simulink model "ADU_Integration_Y2016_simulation"  (R2016b)
settings: Solver=FixedStepDiscrete  StartTime=240  StopTime=300  FixedStep=0.01  RelTol=1e-3  EnableMultiTasking=on
PostLoadFcn:
  | , if any(exist('dsrtsu_mdlpostloadfcn', 'file') == [2, 3, 6]), try dsrtsu_mdlpostloadfcn('Execute', bdroot); catch fprintf('Error in PostLoadFcn (dsrtsu_mdlpostloadfcn) for model "%s":\n %s\n', bdroot, lasterr); end, end,
InitFcn:
  | load 'data/chi2_dat';
  | load 'data/innerLine_struct';
  | load 'data/middleLine_struct';
  | load 'data/outerLine_struct';
  | load 'data/innerLine';
  | load 'data/middleLine';
  | load 'data/outerLine';
  | load 'data/landmarks_patac_schimmel_ccw';
  | load 'data/patac_navi_array';
  | load 'data/sensor';
  | load 'data/map_struct';
  | addpath map_src
  | Integration_Parameter;
  | load 'TestData_001';
values from neighbouring files (symbols this model uses):
  TestData_001 =     [TestData_001.mat]
undefined symbols (not defined in the file or in its folder): a, chi2_dat, innerLine, landmarks_patac_schimmel_ccw, middleLine, outerLine, patac_navi_array, StartNum
libraries: simulink x36, rtican x1
(part 19 of 20)

== matlab function ADU_Integration_Y2016_simulation/Path_Plan1/LaneChangePathPlanningModule1/PathCreator/PathCreator ==
  data: xoptres output; Info_FdIn input; Info_FoIn input; Info_LdIn input; Info_LoIn input; Info_MeIn input; PlanRes output; Tc data_store_memory; V_me data_store_memory; V data_store_memory; L_veh data_store_memory; X_me data_store_memory; X data_store_memory; L_me data_store_memory; T_adj data_store_memory; H data_store_memory; AngleTC data_store_memory; Y data_store_memory; W_veh data_store_memory; Y_me data_store_memory; W_me data_store_memory; Aylimit data_store_memory; Axlimit data_store_memory; X_melimit data_store_memory; k_maxlimit data_store_memory; MSS data_store_memory; DeltaTemp data_store_memory; ArclengthTol data_store_memory; x_qitemp data_store_memory; y_qitemp data_store_memory; theta_qitemp data_store_memory; k_localmaxTemp data_store_memory; ploten data_store_memory; ratio data_store_memory; N_Sample data_store_memory; quadcosu2tbl data_store_memory; quadsinu2tbl data_store_memory; x_inIn input; y_inIn input; angle_inIn input; y_outIn input; angle_outIn input; T_lat data_store_memory; x_in data_store_memory; y_in data_store_memory; angle_in data_store_memory; angle_out data_store_memory; y_out data_store_memory; KurMax output; TrigFlg input; X_melimit_In input; N input; Nlimit data_store_memory; RunCnt data_store_memory; N2 input; Nlimit2 data_store_memory
function [xoptres,PlanRes,KurMax] = PathCreatorFcn(Info_FdIn,Info_FoIn,Info_LdIn,Info_LoIn,Info_MeIn,x_inIn,y_inIn,angle_inIn,y_outIn,angle_outIn,TrigFlg,X_melimit_In,N,N2)
%     global Aylimit Axlimit X_melimit k_maxlimit Tc V L_veh  X L_me T_adj H AngleTC  Y W_veh  W_me X_me MSS x_qitemp y_qitemp theta_qitemp;
    global T_lat V_me DeltaTemp ArclengthTol k_localmaxTemp Nlimit Nlimit2 
    persistent TrigCnt FinishFlg
    if isempty(TrigCnt)
        TrigCnt = 0;
    end
    if isempty(FinishFlg)
        FinishFlg = 1;
    end    
    Nlimit = N;
    Nlimit2 = N2;

    xoptres = [0 0 0]';PlanRes = 0; KurMax = 0;T_long = 4; 
    PreGlbVal(x_inIn,y_inIn,angle_inIn,y_outIn,angle_outIn,Info_FdIn,Info_FoIn,Info_LdIn,Info_LoIn,Info_MeIn,X_melimit_In);
    %Edge Trigger
    if (TrigFlg > 1e-1)
        FinishFlg = 0;
    end
    if FinishFlg == 0
        LB = [10,0.1,5];UB = [40,0.5,20];x0 = [20,0.4,10];
        TrigCnt = 1;
        [xoptres,Res,Sts] = SQPCal(x0',LB',UB',TrigCnt);
        if Sts == 1
            FinishFlg = 1;
            if Res == 1
                PlanRes = 1;  TrigCnt = 0;
%                 x_out=xoptres(1);
%                 V_tar=xoptres(3);
%                 S_arc = ArclengthTol(1) + ArclengthTol(2);    
%                 T_long=xoptres(2)*2*S_arc/(V_tar + V_me);
%                 S_acc = (V_tar + V_me)/2 * T_long;
%                 S_arc = ArclengthTol(1) + ArclengthTol(2);
%                 if S_acc < S_arc
%                     T_lat = T_long + (S_arc - S_acc) / V_tar;
%                 else
%                     a = (V_tar - V_me)/T_long;
%                     V_end = sqrt(V_me^2 + 2*a*S_arc);
%                     if a == 0
%                         T_lat = S_arc / V_me;
%                     else        
%                         T_lat = (V_end - V_me)/a;
%                     end
%                 end 
%                 [ x_qi,y_qi,theta_qi ] = qiConfigCal( x_inIn,y_inIn,angle_inIn,x_out,y_outIn,angle_outIn );
%                 [DeltaTemp(1),k_localmaxTemp(1),ArclengthTol(1)] = ElementaryPathPlot( x_inIn,y_inIn,angle_inIn,x_qi,y_qi,theta_qi );
%                 [DeltaTemp(2),k_localmaxTemp(2),ArclengthTol(2)] = ElementaryPathPlot( x_qi,y_qi,theta_qi,x_out,y_outIn,angle_outIn );
                KurMax = max(k_localmaxTemp);
            end
        else
            TrigCnt = TrigCnt + 1;
        end
    end  
end

function [xoptim,Res,Sts] = SQPCal(x0,LB,UB,Trig)

    global ratio
    global Nlimit Nlimit2
    persistent FinishFlg Pdk PLamda Px1 PCostGTemp PConGTemp StepTrigFlg RunCnt PHk PBk PCurStep PCostG PConG PHx 
    if isempty(RunCnt)
        RunCnt = 0;
    end
    if isempty(PHk)   
        PHk = eye(3);
    end
    if isempty(PBk)   
        PBk = eye(3);
    end    
    if isempty(FinishFlg)
        FinishFlg = 0;
    end
    if isempty(Pdk)
        Pdk = [1 1 1]';
    end
    if isempty(PLamda)
        PLamda = ones(14,1);
    end
    if isempty(Px1)
        Px1 = x0;
    end
    if isempty(PCostGTemp)
        PCostGTemp = zeros(3,1);
    end
    if isempty(PConGTemp)
        PConGTemp = zeros(3,14);
    end
    if isempty(StepTrigFlg)
        StepTrigFlg = 0;
    end
    if isempty(PCurStep)
        % 1 golden 2 qpsub
        PCurStep = 1;
    end
    if isempty(PCostG)
        PCostG = zeros(3,1);
    end
    if isempty(PConG)
        PConG = zeros(3,14);
    end
    if isempty(PHx)
        PHx = zeros(1,14);
    end
    ratio = 1e3;
    limit1 = [0 0 0];limit2 = [0 0 0];lolimit = [0 0 0];hilimit = [0 0 0]; Alpha = 1;
    dk = [1 1 1]'; Lamda = ones(14,1);  x1 = x0;Bk=eye(3);Hk=eye(3);xoptim = x0;; CostGTemp = zeros(3,1);ConGTemp = zeros(3,14);Sts = 0;Res = 0;CostG = zeros(3,1);ConG = zeros(3,14);Hx = zeros(1,14);
%     while (1)
    if PCurStep == 1
        if (RunCnt == 0)
            if Trig == 1
                %First Trig 
                RunCnt = RunCnt + 1;
                FinishFlg = 0;
                [CostG,ConG,Costx,Hx]=GradientCal(x0,LB,UB);
                CostGTemp = CostG;
                ConGTemp = ConG;
            end
        else
            %LoadFrom Previous Step
            dk = Pdk;Lamda = PLamda;x1 = Px1;CostGTemp = PCostGTemp;ConGTemp = PConGTemp;Hk = PHk;Bk = PBk;
            for i = 1:3
                if abs(dk(i)) < 1e-4
                    limit1(i) = 0;
                    limit2(i) = 1e4;                
                else
                    limit1(i) = ((LB(i) - x1(i))./dk(i));
                    limit2(i) = ((UB(i) - x1(i))./dk(i));
                end
                lolimit(i) = min([limit1(i),limit2(i)]);
                hilimit(i) = max([limit1(i),limit2(i)]);
            end
            Lo = max([lolimit,0]);
            Hi = min(hilimit);
            if (Hi <0)||(Hi < Lo)
                FinishFlg = 1;
            end
            Accurcy = min(abs([1e-2/dk(1),1e-3/dk(2),1e-2/dk(3)]));
            Alpha=goldenSearch(x1,dk,Lo,Hi,LB,UB,Accurcy);
            if max(abs(Alpha * dk)) < 1e-3
                FinishFlg = 1;
            end
            BestStep = Alpha * dk;
            if (BestStep(1) < 1e-2)&& (BestStep(3) < 1e-2) && (BestStep(2) < 1e-3)                          
            end
            x1temp = x1;
            x1 = x1 + Alpha * dk;
            sk=x1-x1temp; 
            [CostG,ConG,Costx,Hx] = GradientCal(x1,LB,UB);
            initial_CostGLx = LxGradientCal(CostGTemp,ConGTemp,Lamda);
            CostGLx = LxGradientCal(CostG,ConG,Lamda);
            CostGTemp = CostG;
            ConGTemp = ConG;
            yk = CostGLx-initial_CostGLx; 
            if  yk'*sk>0
                Bk=Bk+(sk*sk')/(yk'*sk)-(Bk*yk*yk'*Bk)/(yk'*Bk*yk);  
            else 
            end
            if yk'* sk > 0 
                Hk = Hk + ((sk - Hk*yk)*sk' + sk*(sk-Hk*yk)')/(yk'*sk)-(sk-Hk*yk)'*yk*sk*sk'/(yk'*sk)^2;
            end
        end
        PHk = Hk;PCostG = CostG;PConG = ConG;PHx = Hx;Px1 = x1;PConGTemp = ConGTemp;PBk = Bk;PCostGTemp = CostGTemp; 
        PCurStep = 2;
    else          
        if (FinishFlg == 0)&&(PCurStep == 2)
            Hk = PHk;CostG = PCostG;ConG = PConG;Hx = PHx;PCurStep = 1;
            y1 = ones(14,1);w1 = ones(14,1);dx1 = ones(3,1);
            [dk,Lamda] = qpfunc( Hk,CostG,ConG',-Hx,dx1,y1,w1 );  
            if (norm(dk,2)<1e-3)||(Alpha < 1e-4)
                FinishFlg = 1;
            else
                Pdk = dk; PLamda = Lamda; 
            end
        end
        PCurStep = 1; 
    end
    RunCnt = RunCnt + 1;
    if RunCnt > Nlimit
        FinishFlg = 1;
    end
    if FinishFlg == 1;        
        Sts = 1;
        if RunCnt > Nlimit
            % 0 Failure 1 Success
           Res = 0;
        else
           Res = 1;
           xoptim = Px1; 
        end
        RunCnt = 0;PCurStep = 1;
    end
end

function [CostG,ConG,Costx,Hx]= GradientCal(Xin,LB,UB)

value1Cost=ones(3,1);
value2Cost=ones(3,1);
value1Con=ones(3,14);
value2Con=ones(3,14);

dx=1e-1;
dy=1e-1;
dz=1e-1;
Xin_x=Xin+ [dx;0;0];
Xin_y=Xin+ [0;dy;0];
Xin_z=Xin+ [0;0;dz];
value1Cost(1) = (  CostFun(Xin_x) - CostFun(Xin) ) / dx;    %x
value1Cost(2) = (  CostFun(Xin_y) - CostFun(Xin) ) / dy ;   %y
value1Cost(3) = (  CostFun(Xin_z) - CostFun(Xin) ) / dz ;   %z
ConFuncXinVal = ConFunc(Xin,LB,UB);
value1Con(1,:) = (  ConFunc(Xin_x,LB,UB) - ConFuncXinVal ) / dx;    %x
value1Con(2,:) = (  ConFunc(Xin_y,LB,UB) - ConFuncXinVal ) / dy ;   %y
value1Con(3,:) = (  ConFunc(Xin_z,LB,UB) - ConFuncXinVal ) / dz ;   %z
CostG = value1Cost;
ConG = value1Con;
Costx = CostFun(Xin);
Hx = ConFuncXinVal;

end

function bestStep=goldenSearch(x0,direction,lo,hi,LB,UB,Accurcy)
    global Nlimit 
    a=lo;
    b=hi;
    % TBD Change 2
    error=1e-2;
    error = Accurcy;
    golden=0.61803398;
    goldenn = 0;
    alpha=a + (1-golden) * (b-a);
    beta=a + golden * (b-a);
    f_alpha=Pfunc( x0 + alpha * direction,LB,UB);
    f_beta=Pfunc( x0 + beta * direction,LB,UB);

    while(abs(b-a)>error)

    %     a1=a;  b1=b;
        goldenn = goldenn + 1;
        b - a;
        f_beta - f_alpha;
        if alpha>beta
    %         a=a1;b=b1;
            alpha=a + (1-golden) * (b-a);
            beta=a + golden * (b-a);
            f_alpha=Pfunc( x0 + alpha * direction,LB,UB);
            f_beta=Pfunc( x0 + beta * direction,LB,UB);       
        end  
        if f_alpha<=f_beta
            b=beta;
            beta=alpha;
            f_beta=f_alpha;
            alpha=a + (b-beta);
            f_alpha=Pfunc( x0 + alpha*direction,LB,UB);
    %         a1=a;  b1=b;
        else
            a = alpha;
            alpha = beta;
            f_alpha = f_beta;
            beta = b - (alpha-a);
            f_beta = Pfunc( x0 + beta * direction,LB,UB);
    %         a1=a;  b1=b;
        end
        if goldenn > Nlimit
            break;
        end

    end

    if Pfunc(x0 + a * direction,LB,UB)<Pfunc(x0 + b * direction,LB,UB)
        bestStep=a;
    else
        bestStep=b;
    end
    n = 0;
    goldenn
end

function [dk,dkLamda] = qpfunc( H,c,A,b,x1,y1,w1 )
%UNTITLED2 Summary of this function goes here
%   Detailed explanation goes here
    global Nlimit 
Delta = 0.1;
P = 0.9;
E = ones(length(y1),1);
m = length(b);
qpfunck = 0;

    while(1)

        qpfunck = qpfunck+1;
        if qpfunck > Nlimit
            dk = x1;
            dkLamda = y1;
            break;
        end
        Y = diag(y1);
        W = diag(w1);
        Rho = b - A*x1 + w1;
        Sigma = c + H*x1 -A'*y1;
        Gamma = y1'*w1;
        Mu = Delta * Gamma / m;
        newMatricL = [-H A';A inv(Y)*W];
        newMatricR = [c + H*x1 - A'*y1;b-A*x1 + Mu*inv(Y)*E];
        dxy = inv(newMatricL)*newMatricR;
        dx = dxy(1:length(x1));
        dy = dxy((length(x1)+1):(length(dxy)));
        dw = inv(Y)*(Mu*E - Y*W*E - W*dy);
        LamdaTemp1 = [-dy./y1,-dw./w1];
        Lamda = min([1, P*pinv(max([-dy./y1;-dw./w1]))]);
        if (norm(Gamma,1)<1e-3)&(norm(Rho,1)<1e-3)&(norm(Sigma,1)<1e-3)
            dk = x1;
            dkLamda = y1;
            break;
        else
            x1 = x1 + Lamda*dx;
            y1 = y1 + Lamda*dy;
            w1 = w1 + Lamda*dw;
        end
    end
    qpfunck;
end

function dLxVal= LxGradientCal2(Xin,Lamda,LB,UB,CostGTemp,ConGTemp)

    value1=ones(3,1);
    value2=ones(3,1);
    value1LxVal = [0 0 0];
    value2LxVal = [0 0 0];
    dx=1e-1;
    dy=1e-1;
    dz=1e-1;
    Xin_x=Xin+ [dx;0;0];
    Xin_y=Xin+ [0;dy;0];
    Xin_z=Xin+ [0;0;dz];

    ConFuncValue = ConFunc(Xin,LB,UB);

    value1LxVal(1) = (CostFun(Xin_x) - CostFun(Xin)- Lamda' *  ConFunc(Xin_x,LB,UB) + Lamda' *  ConFuncValue)/dx;
    value1LxVal(2) = (CostFun(Xin_y) - CostFun(Xin)- Lamda' *  ConFunc(Xin_y,LB,UB) + Lamda' *  ConFuncValue)/dy;
    value1LxVal(3) = (CostFun(Xin_z) - CostFun(Xin)- Lamda' *  ConFunc(Xin_z,LB,UB) + Lamda' *  ConFuncValue)/dz;

    dLxVal = value1LxVal;
    dLxVal = dLxVal';
    
end
% TBD change 5

function dLxVal= LxGradientCal(CostG,ConG,Lamda)

    dLxVal = CostG -  ConG* Lamda;
    
end

function Pval= Pfunc(Xin,LB,UB)
    global ratio   
    [C,Ceq] = LaneChgNonLinearCon( Xin);
    LengthC = 8;
    LengthLB = length(LB);
    C((LengthC+1):(LengthC+LengthLB))= Xin - UB;
    C((LengthC+LengthLB+1):(LengthC+LengthLB+LengthLB))= LB - Xin;

    hminx= min([0,min(-C)]);
    Pval = - Xin(3) + ratio* norm(hminx,1);
end

function Fcost= CostFun(Xin)

    Fcost = LaneChgCostFunc(Xin);

end

function ConVal= ConFunc(Xin,LB,UB)
    [C,Ceq] = LaneChgNonLinearCon( Xin);

    LengthC = 8;
    LengthLB = length(LB);
    C((LengthC+1):(LengthC+LengthLB))= Xin - UB;
    C((LengthC+LengthLB+1):(LengthC+LengthLB+LengthLB))= LB - Xin;
    C=-C;
    ConVal = C;

end
function CosFunValue = LaneChgCostFunc(Xin)
    CosFunValue = -Xin(3);
end
function [ C,Ceq ] = LaneChgNonLinearCon( Xin )
global V_me V L_veh X_me X L_me T_adj ;
global Aylimit  X_melimit k_maxlimit;
% global T_lat Axlimit 
global DeltaTemp k_localmaxTemp ArclengthTol
global x_qitemp y_qitemp theta_qitemp
global x_in y_in angle_in y_out angle_out 
C = zeros(14,1);
Tc = [0 0 0 0]';
MSS = [0 0 0 0]';
%T_long=Xin(2);
V_tar=Xin(3);

T_lat = 5;
% x_in = 0;y_in = 0;angle_in = 0;y_out = 3;angle_out = 0;
x_out = Xin(1);
[ x_qi,y_qi,theta_qi ] = qiConfigCal( x_in,y_in,angle_in,x_out,y_out,angle_out );
 x_qitemp = x_qi;y_qitemp=y_qi;theta_qitemp=theta_qi;
%[ x_qitemp,y_qitemp,theta_qitemp ] = qiConfigCal( x_in,y_in,angle_in,x_out,y_out,angle_out );
[DeltaTemp(1),k_localmaxTemp(1),ArclengthTol(1)] = ElementaryPathPlot( x_in,y_in,angle_in,x_qi,y_qi,theta_qi );
[DeltaTemp(2),k_localmaxTemp(2),ArclengthTol(2)] = ElementaryPathPlot( x_qi,y_qi,theta_qi,x_out,y_out,angle_out );
Ycal = [1.5,1.5];
% 1 Fl 2 Rr
[xposition,yposition,Theta,ArcPos] = ArcPosCal( angle_out,angle_in,x_in,y_in,x_out,y_out,Ycal );
%Fd
Tc(1) = (xposition(1) - X(1))/(V(1)+1e-6);
Tc(2) = (xposition(2) - X(2))/(V(2)+1e-6);
Tc(3) = (xposition(1) - X(3))/(V(3)+1e-6);
Tc(4) = (xposition(2) - X(4))/(V(4)+1e-6);
for i = 1:4
    if Tc(i) < 0
        Tc(i) = 0;
    else
    end
end
        
delta_limit = 0.5;
DeltalimitC = max(abs(DeltaTemp)) - delta_limit;
AylimitC = max(abs(k_localmaxTemp)) * V_tar^2 - Aylimit;
KmlimitC = max(abs(k_localmaxTemp)) - k_maxlimit;

S_arc = ArclengthTol(1) + ArclengthTol(2);
if V_tar == V_me
    T_lat = S_arc / V_me;
    T_long = 0;
else
    Tuplimit = 2 * S_arc / (V_tar + V_me);
    T_long = Tuplimit * Xin(2);
    S_acc = (V_tar + V_me)/2 * T_long;
    if S_acc < S_arc
        T_lat = T_long + (S_arc - S_acc) / V_tar;
    else
        a = (V_tar - V_me)/T_long;
        V_end = sqrt(V_me^2 + 2*a*S_arc);
        if a == 0
            T_lat = S_arc / V_me;
        else        
            T_lat = (V_end - V_me)/a;
        end
    end
end
%MSSFdlimitC < 0 which means safemargin >0
MSS(1) = MSSFdJudgment( V_tar,V_me,V(1),T_lat,Tc(1),T_lat,T_adj );
MSS(2) = MSSFoJudgment( V_tar,V_me,V(2),T_lat,Tc(2),T_lat,T_adj );
MSS(3) = MSSLdJudgment( V_tar,V_me,V(3),T_lat,Tc(3),T_lat,T_adj );
MSS(4) = MSSLoJudgment( V_tar,V_me,V(4),T_lat,Tc(4),T_lat,T_adj );
X_meTemp = X_me - 2 * (ArcPos(1)+ArcPos(2) - xposition(1) - xposition(2));
MSSFdlimitC = X(1) - X_meTemp + L_me + MSS(1);
MSSFolimitC = X(2) - X_meTemp + L_me + MSS(2);
MSSLdlimitC = MSS(3) + X_meTemp + L_veh(3) - X(3);
MSSLolimitC = MSS(4) + X_meTemp + L_veh(4) - X(4);
X_melimitC =  2 * x_out - X_melimit;

C(1)=DeltalimitC;
C(2)=KmlimitC;
C(3)=MSSFdlimitC;
C(4)=MSSFolimitC;
C(5)=MSSLdlimitC;
C(6)=MSSLolimitC;
C(7)=X_melimitC;
C(8)=AylimitC; 

Ceq = [];

end

function [xposition,yposition,Theta,ArcPos] = ArcPosCal( angle_out,angle_in,x_in,y_in,x_out,y_out,Ycal )
%UNTITLED2 Summary of this function goes here
%   Detailed explanation goes here
    global  ArclengthTol
%     global x_qitemp y_qitemp theta_qitemp k_localmaxTemp DeltaTemp
    xposition = [0 0];
    yposition = [1.5 1.5];
    Theta = [0 0 ];
    ArcPos = [0 0];
    [ArcPos,xposition,Theta] = SecantMethod2( angle_out,angle_in,x_in,y_in,x_out,y_out,0.8*ArclengthTol(1),1.1*ArclengthTol(1) ); 
end
 
% end
function [xres,xposition,theta] = SecantMethod2( angle_out,angle_in,x_in,y_in,x_out,y_out,x0,x1 )
    xres = [0 0 ];
    temp1 = x0;
    temp2 = x1;
    xposition = [0 0];
    theta = [0 0]; 
    [xpositionFl1,ypositionFl1,ThetaFl1] = LaneChgFlPosCal2( x1,angle_out,angle_in,x_in,y_in,x_out,y_out );
    funx1 = ypositionFl1 - 1.5;
    [xpositionFl0,ypositionFl0,ThetaFl0] = LaneChgFlPosCal2( x0,angle_out,angle_in,x_in,y_in,x_out,y_out );
    funx0 = ypositionFl0 - 1.5;
    x2 = x1-funx1*(x1-x0)/(funx1-funx0);
    %x2 = x1-fun(x1)*(x1-x0)/(fun(x1)-fun(x0));
    Secantn = 1;
    while (abs(x1-x0)>=1.0e-1) && (Secantn<=20)      %
        x0=x1;                                       %x1x0
        x1=x2;                                       %x2x1
        %x2=x1-fun(x1)*(x1-x0)/(fun(x1)-fun(x0));     %
        [xpositionFl1,ypositionFl1,ThetaFl1] = LaneChgFlPosCal2( x1,angle_out,angle_in,x_in,y_in,x_out,y_out );
        funx1 = ypositionFl1 - 1.5;
        [xpositionFl0,ypositionFl0,ThetaFl0] = LaneChgFlPosCal2( x0,angle_out,angle_in,x_in,y_in,x_out,y_out );
        funx0 = ypositionFl0 - 1.5;
        x2 = x1-funx1*(x1-x0)/(funx1-funx0);
        Secantn=Secantn+1;
    end
    Secantn
    xres(1) = x2;
    xposition(1) = (xpositionFl1 + xpositionFl0) /2;
    theta(1) = (ThetaFl1 + ThetaFl0)/2;
    % TBD change 4
%     x0 = x2;
    x0 = temp1;
    x1 = temp2;
    [xpositionRr1,ypositionRr1,ThetaRr1] = LaneChgRrPosCal2( x1,angle_out,angle_in,x_in,y_in,x_out,y_out );
    funx1 = ypositionRr1 - 1.5;
    [xpositionRr0,ypositionRr0,ThetaRr0] = LaneChgRrPosCal2( x0,angle_out,angle_in,x_in,y_in,x_out,y_out );
    funx0 = ypositionRr0 - 1.5;
    x2 = x1-funx1*(x1-x0)/(funx1-funx0);
    %x2 = x1-fun(x1)*(x1-x0)/(fun(x1)-fun(x0));    n = 1;
    Secantn = 0;
    while (abs(x1-x0)>=1.0e-1) && (Secantn<=20)      %
        x0=x1;                                       %x1x0
        x1=x2;                                       %x2x1
        %x2=x1-fun(x1)*(x1-x0)/(fun(x1)-fun(x0));     %
        [xpositionRr1,ypositionRr1,ThetaRr1] = LaneChgRrPosCal2( x1,angle_out,angle_in,x_in,y_in,x_out,y_out );
        funx1 = ypositionRr1 - 1.5;
        [xpositionRr0,ypositionRr0,ThetaRr0] = LaneChgRrPosCal2( x0,angle_out,angle_in,x_in,y_in,x_out,y_out );
        funx0 = ypositionRr0 - 1.5;
        x2 = x1-funx1*(x1-x0)/(funx1-funx0);
        Secantn=Secantn+1;
    end
    Secantn
    xres(2) = x2;
    xposition(2) = (xpositionRr1 + xpositionRr0) /2;
    theta(2) = (ThetaRr1 + ThetaRr0)/2;
end
function xres = SecantMethod( angle_out,angle_in,x_in,y_in,x_out,y_out,x0,x1 )
%UNTITLED2 Summary of this function goes here
%   Detailed explanation goes here
%     global DeltaTemp ArclengthTol
%     global x_qitemp y_qitemp theta_qitemp k_localmaxTemp    
    xres = [0 0 ];
    temp1 = x0;
    temp2 = x1;
    funx1 = LaneChgFlPosCal( x1,angle_out,angle_in,x_in,y_in,x_out,y_out ) - 1.5;
    funx0 = LaneChgFlPosCal( x0,angle_out,angle_in,x_in,y_in,x_out,y_out ) - 1.5;
    x2 = x1-funx1*(x1-x0)/(funx1-funx0);
    %x2 = x1-fun(x1)*(x1-x0)/(fun(x1)-fun(x0));
    Secantn = 1;
    while (abs(x1-x0)>=1.0e-1) && (Secantn<=20)      %
        x0=x1;                                       %x1x0
        x1=x2;                                       %x2x1
        %x2=x1-fun(x1)*(x1-x0)/(fun(x1)-fun(x0));     %
        funx1 = LaneChgFlPosCal( x1,angle_out,angle_in,x_in,y_in,x_out,y_out ) - 1.5;
        funx0 = LaneChgFlPosCal( x0,angle_out,angle_in,x_in,y_in,x_out,y_out ) - 1.5;
        x2 = x1-funx1*(x1-x0)/(funx1-funx0);
        Secantn=Secantn+1;
    end
    Secantn
    xres(1) = x2;

    % TBD change 4
%     x0 = x2;
    x0 = temp1;
    x1 = temp2;
    funx1 = LaneChgRrPosCal( x1,angle_out,angle_in,x_in,y_in,x_out,y_out ) - 1.5;
    funx0 = LaneChgRrPosCal( x0,angle_out,angle_in,x_in,y_in,x_out,y_out ) - 1.5;
    x2 = x1-funx1*(x1-x0)/(funx1-funx0);
    %x2 = x1-fun(x1)*(x1-x0)/(fun(x1)-fun(x0));    n = 1;
    Secantn = 0;
    while (abs(x1-x0)>=1.0e-1) && (Secantn<=20)      %
        x0=x1;                                       %x1x0
        x1=x2;                                       %x2x1
        %x2=x1-fun(x1)*(x1-x0)/(fun(x1)-fun(x0));     %
        funx1 = LaneChgRrPosCal( x1,angle_out,angle_in,x_in,y_in,x_out,y_out ) - 1.5;
        funx0 = LaneChgRrPosCal( x0,angle_out,angle_in,x_in,y_in,x_out,y_out ) - 1.5;
        x2 = x1-funx1*(x1-x0)/(funx1-funx0);
        Secantn=Secantn+1;
    end
    Secantn
    xres(2) = x2;
end
function ypositionRr = LaneChgRrPosCal( Arc,angle_out,angle_in,x_in,y_in,x_out,y_out )
%UNTITLED3 Summary of this function goes here
%   Detailed explanation goes here
    global DeltaTemp ArclengthTol
    global x_qitemp y_qitemp theta_qitemp
    global L_me W_me
    if Arc <= ArclengthTol(1)
        [xposition,yposition,Theta] = ElementaryPosCal( Arc,DeltaTemp(1),ArclengthTol(1),theta_qitemp,angle_in,x_in,y_in,x_qitemp,y_qitemp );
    else
       Arc = Arc - ArclengthTol(1);
        [xposition,yposition,Theta] = ElementaryPosCal( Arc,DeltaTemp(2),ArclengthTol(2),angle_out,theta_qitemp,x_qitemp,y_qitemp,x_out,y_out );
    end
    xpositionRr = xposition + W_me * sin(Theta) / 2;
    ypositionRr = yposition - W_me * cos(Theta) / 2;
end

function ypositionFl = LaneChgFlPosCal( Arc,angle_out,angle_in,x_in,y_in,x_out,y_out )
%UNTITLED3 Summary of this function goes here
%   Detailed explanation goes here
    global DeltaTemp ArclengthTol
    global x_qitemp y_qitemp theta_qitemp
    global L_me W_me
    if Arc <= ArclengthTol(1)
        [xposition,yposition,Theta] = ElementaryPosCal( Arc,DeltaTemp(1),ArclengthTol(1),theta_qitemp,angle_in,x_in,y_in,x_qitemp,y_qitemp );
    else
       Arc = Arc - ArclengthTol(1);
        [xposition,yposition,Theta] = ElementaryPosCal( Arc,DeltaTemp(2),ArclengthTol(2),angle_out,theta_qitemp,x_qitemp,y_qitemp,x_out,y_out );
    end
    xpositionFl = xposition + L_me * cos(Theta) - W_me * sin(Theta) / 2;
    ypositionFl = yposition + L_me * sin(Theta) + W_me * cos(Theta) / 2;
end

function [xpositionFl,ypositionFl,Theta] = LaneChgFlPosCal2( Arc,angle_out,angle_in,x_in,y_in,x_out,y_out )
%UNTITLED3 Summary of this function goes here
%   Detailed explanation goes here
    global DeltaTemp ArclengthTol
    global x_qitemp y_qitemp theta_qitemp
    global L_me W_me
    if Arc <= ArclengthTol(1)
        [xposition,yposition,Theta] = ElementaryPosCal( Arc,DeltaTemp(1),ArclengthTol(1),theta_qitemp,angle_in,x_in,y_in,x_qitemp,y_qitemp );
    else
       Arc = Arc - ArclengthTol(1);
        [xposition,yposition,Theta] = ElementaryPosCal( Arc,DeltaTemp(2),ArclengthTol(2),angle_out,theta_qitemp,x_qitemp,y_qitemp,x_out,y_out );
    end
    xpositionFl = xposition + L_me * cos(Theta) - W_me * sin(Theta) / 2;
    ypositionFl = yposition + L_me * sin(Theta) + W_me * cos(Theta) / 2;
end

function [xpositionRr,ypositionRr,Theta] = LaneChgRrPosCal2( Arc,angle_out,angle_in,x_in,y_in,x_out,y_out )
%UNTITLED3 Summary of this function goes here
%   Detailed explanation goes here
    global DeltaTemp ArclengthTol
    global x_qitemp y_qitemp theta_qitemp
    global L_me W_me
    if Arc <= ArclengthTol(1)
        [xposition,yposition,Theta] = ElementaryPosCal( Arc,DeltaTemp(1),ArclengthTol(1),theta_qitemp,angle_in,x_in,y_in,x_qitemp,y_qitemp );
    else
       Arc = Arc - ArclengthTol(1);
        [xposition,yposition,Theta] = ElementaryPosCal( Arc,DeltaTemp(2),ArclengthTol(2),angle_out,theta_qitemp,x_qitemp,y_qitemp,x_out,y_out );
    end
    xpositionRr = xposition + W_me * sin(Theta) / 2;
    ypositionRr = yposition - W_me * cos(Theta) / 2;
end

function [xposition,yposition,Theta] = ElementaryPosCal( Arc,Delta,Arclength,angle_out,angle_in,x_in,y_in,x_out,y_out )
%UNTITLED Summary of this function goes here
%   Detailed explanation goes here   
    Beta = (angle_out - angle_in)/2;
    theta_rot = angle_in;
    x_outRot = (x_out - x_in)*cos(theta_rot) + (y_out - y_in)*sin(theta_rot);
    y_outRot = (y_out - y_in)*cos(theta_rot) - (x_out - x_in)*sin(theta_rot);    
    if Beta == 0
        SignBeta = 1;
    else
        SignBeta = sign(Beta);
    end
    if Arc < Arclength/2    
        ulimit = Arc * sqrt(abs( Delta )/2);
        Theta = Delta * (Arc)^2/2;
        xpositionTemp = sqrt(2/abs(Delta))*quadcosu2(ulimit);
        ypositionTemp = sqrt(2/abs(Delta))*quadsinu2(ulimit) * SignBeta;
    else
        ulimit = (Arclength - Arc) * sqrt(abs(Delta)/2); 
        %Theta = 2*Beta*SignBeta - Delta * (Arclength - Arc)^2/2; 
        xpositionMirrTemp = sqrt(2/abs(Delta))*quadcosu2(ulimit);
        ypositionMirrTemp = sqrt(2/abs(Delta))*quadsinu2(ulimit) * SignBeta;
        %mirror line Ax+By+C=0
        x_mirr = (x_outRot)/2;
        y_mirr = (y_outRot)/2;
        angle_mirr = pi/2 + atan((y_outRot)/(x_outRot));
        A = tan(angle_mirr);
        B = -1;
        C = y_mirr - A * x_mirr;      
        %two points are symmetrical to the Ax+By+C we just defined
        xpositionTemp = xpositionMirrTemp - 2*A*(A*xpositionMirrTemp+B*ypositionMirrTemp+C)/(A^2+B^2);
        ypositionTemp = ypositionMirrTemp - 2*B*(A*xpositionMirrTemp+B*ypositionMirrTemp+C)/(A^2+B^2);
        Theta = 2*abs(Beta)*SignBeta - Delta * (Arclength - Arc)^2/2;          
    end
    theta_rot = - angle_in;   
    xposition = xpositionTemp*cos(theta_rot) + ypositionTemp*sin(theta_rot);
    yposition = ypositionTemp*cos(theta_rot) - xpositionTemp*sin(theta_rot) ;  
    xposition = xposition + x_in;
    yposition = yposition + y_in;
    Theta = Theta + angle_in;    
end

function [ x_qi,y_qi,theta_qi ] = qiConfigCal( x_in,y_in,angle_in,x_out,y_out,angle_out )
%UNTITLED2 Summary of this function goes here
%   Detailed explanation goes here
    kesi_en = angle_out - angle_in;
    r_en = sqrt((x_in-x_out)^2+(y_in-y_out)^2);
    k_qi_en = 2 * sin(kesi_en/2)/r_en;    
    if k_qi_en == 0
        x_qi = (x_in + x_out)/2;
        y_qi = (y_in + y_out)/2;
        theta_qi = asin((y_out - y_in)/r_en) * 2 + (angle_in + angle_out)/2;        
    else
        r_qi_en = abs(1/k_qi_en);
        angle_qi_CC = 2* asin(r_en*k_qi_en/2);
        alpha_en = atan((y_out-y_in)/(x_out-x_in));
        if (x_out < x_in)
            alpha_en = alpha_en + pi;
        elseif angle_in > pi
            alpha_en = alpha_en + pi*2;
        end
        if alpha_en > 1e-5
            while alpha_en > 2*pi
                alpha_en = alpha_en - 2 * pi;
            end
        else
            while alpha_en < -2*pi
                alpha_en = alpha_en + 2*pi;
            end
        end

        angle_qi = angle_qi_CC/2;
        if k_qi_en == 0
            signK = 1;
        else
            signK = sign(k_qi_en);
        end
        a = r_qi_en * cos(-angle_qi_CC/2+angle_qi)-sqrt(r_qi_en^2-r_en^2/4);
        b = r_qi_en * sin(-angle_qi_CC/2+angle_qi);
        x_qi = a * sin(alpha_en) * signK - b * cos(alpha_en) * signK + (x_in + x_out) / 2;
        y_qi = - a * cos(alpha_en) * signK - b * sin(alpha_en) * signK + (y_in + y_out) / 2 ; 
        theta_qi = - ( angle_in +angle_out )/2 + 2 * alpha_en;
    end
    if theta_qi > 1e-5
        while theta_qi > 2*pi
            theta_qi = theta_qi - 2 * pi;
        end
    else
        while theta_qi < -2*pi
            theta_qi = theta_qi + 2*pi;
        end
    end       
end

function [Delta,k_localmax,Arclength] = ElementaryPathPlot( x_in,y_in,angle_in,x_out,y_out,angle_out )
    %UNTITLED2 Summary of this function goes here
    %   Detailed explanation goes here
    Nlen = 20;
    xposition = zeros(Nlen,1);
    yposition = zeros(Nlen,1);
    Theta = zeros(Nlen,1);
    kur = zeros(Nlen,1);
    %ArcPos = zeros(Nlen,1);
    Beta = (angle_out - angle_in)/2;
    r = sqrt((x_in-x_out)^2+(y_in-y_out)^2);
    %Move
    x_inMove = x_in - x_in;
    y_inMove = y_in - y_in;
    x_outMove = x_out - x_in;
    y_outMove = y_out - y_in;
    %Rotate
    theta_rot = angle_in;
    x_inRot = x_inMove*cos(theta_rot) + y_inMove*sin(theta_rot);
    x_outRot = x_outMove*cos(theta_rot) + y_outMove*sin(theta_rot);
    y_inRot = y_inMove*cos(theta_rot) - x_inMove*sin(theta_rot);
    y_outRot = y_outMove*cos(theta_rot) - x_outMove*sin(theta_rot);    
    SignBeta = sign(Beta);
    Beta = abs(Beta);
    ulimit = sqrt(Beta);
    D_BetaVal = sin(Beta)*quadsinu2(ulimit)+cos(Beta)*quadcosu2(ulimit);
    Delta = 8*SignBeta*D_BetaVal^2/r^2;
    %longth of the trajectary     
    Arclength = 2*sqrt(2*abs(Beta/Delta*SignBeta));
    k_localmax = Delta * Arclength/2;    
end

function quadcosu2val = quadcosu2( ulimit )
    %UNTITLED4 Summary of this function goes here
    %   Detailed explanation goes here
    % this function is used to calculate the integral of cos(x^2),which is used
    % to calculate x position
    global quadcosu2tbl
    index = fix(ulimit/0.005) + 1;
    quadcosu2val = quadcosu2tbl(index);
end

function quadsinu2val = quadsinu2( ulimit )
%UNTITLED4 Summary of this function goes here
%   Detailed explanation goes here
% this function is used to calculate the integral of sin(x^2),which is used
% to calculate y position
    global quadsinu2tbl 
    index = fix(ulimit/0.005) + 1;
    quadsinu2val = quadsinu2tbl(index);
end

function MSS = MSSFdJudgment( V_tar,V_me,V_obj,T_long,Tc,T_lat,T_adj )
%UNTITLED5 Summary of this function goes here
%   Detailed explanation goes here
    
    if abs(V_me-V_tar)<1e-5
    
        if V_me>V_obj
            MSS = (-V_me+V_obj)*(Tc+T_adj);
        else
            MSS = (-V_me+V_obj)*(T_adj+T_lat);
        end
        
    else

        T_max = (V_obj - V_me)/(V_tar - V_me)*T_long;
        MSSTemp1 = 0;
        MSSTemp2 = 0;

        if Tc < T_long
            if (V_obj >= V_tar)&&(V_tar >V_me)
                MSS = MSSCalculate( V_tar,V_me,V_obj,T_long,T_lat,0 ,T_adj);
            elseif (V_obj >= V_me)&&(V_me > V_tar)
                MSS = MSSCalculate( V_tar,V_me,V_obj,T_long,T_lat,0 ,T_adj);
            elseif (V_me >= V_obj)&&(V_obj >= V_tar)
                if Tc > T_max
                    MSS = MSSCalculate( V_tar,V_me,V_obj,T_long,T_lat,0 ,T_adj);
                else
                    MSSTemp1 = MSSCalculate( V_tar,V_me,V_obj,T_long,T_lat,0 ,T_adj);  
                    MSSTemp2 = MSSCalculate( V_tar,V_me,V_obj,T_long,Tc,0 ,T_adj);
                    MSS = max(MSSTemp1,MSSTemp2);           
                end

            elseif (V_obj <= V_tar)&&(V_tar < V_me)
                MSS = MSSCalculate( V_tar,V_me,V_obj,T_long,Tc,0 ,T_adj);

            elseif (V_obj <= V_me)&&(V_me < V_tar)
                MSS = MSSCalculate( V_tar,V_me,V_obj,T_long,Tc,0 ,T_adj);

            elseif (V_me <= V_obj)&&(V_obj <= V_tar)
                if Tc > T_max
                    MSS = MSSCalculate( V_tar,V_me,V_obj,T_long,Tc,0 ,T_adj);
                else 
                    MSS = MSSCalculate( V_tar,V_me,V_obj,T_long,T_max,0 ,T_adj);
                end            
            else
                %Nothing
                MSS = 255;
            end    
        else
            % Tc > T_long
            if  V_tar > V_obj
                MSS = MSSCalculate( V_tar,V_me,V_obj,T_long,Tc,0 ,T_adj);
            else
                MSS = MSSCalculate( V_tar,V_me,V_obj,T_long,T_lat,0 ,T_adj);
            end  
        end
    end
    
end

function MSS = MSSFoJudgment( V_tar,V_me,V_obj,T_long,Tc,T_lat,T_adj )
%UNTITLED5 Summary of this function goes here
%   Detailed explanation goes here

    if abs(V_me-V_tar)<1e-5

        if V_me>V_obj
            MSS = 0;
        else
            MSS = (-V_me+V_obj)*(T_adj+Tc);
        end

    else
        T_max = (V_obj - V_me)/(V_tar - V_me)*T_long;
        MSSTemp1 = 0;
        MSSTemp2 = 0;
        if Tc < T_long
            if (V_obj >= V_tar)&&(V_tar >V_me)
                MSS = MSSCalculate( V_tar,V_me,V_obj,T_long,Tc,0 ,T_adj);
            elseif (V_obj >= V_me)&&(V_me >V_tar)
                MSS = MSSCalculate( V_tar,V_me,V_obj,T_long,Tc,0 ,T_adj);
            elseif (V_me >= V_obj)&&(V_obj >= V_tar)
                if Tc > 2*T_max
                    MSS = MSSCalculate( V_tar,V_me,V_obj,T_long,Tc,0 ,T_adj);
                else
                    MSS = 0;           
                end

            elseif (V_obj <= V_tar)&&(V_tar < V_me)
                %MSS = MSSCalculate( V_tar,V_me,V_obj,T_long,0,0 );
                MSS = 0;

            elseif (V_obj <= V_me)&&(V_me < V_tar)
                %MSS = MSSCalculate( V_tar,V_me,V_obj,T_long,0,0 );
                MSS = 0;
            elseif (V_me <= V_obj)&&(V_obj <= V_tar)
                if Tc > T_max
                    MSS = MSSCalculate( V_tar,V_me,V_obj,T_long,T_max,0 ,T_adj);
                else 
                    MSS = MSSCalculate( V_tar,V_me,V_obj,T_long,Tc,0 ,T_adj);
                end            
            else
                %Nothing
                MSS = 255;
            end    
        else
            % Tc > T_long
            if (V_obj >= V_tar)&&(V_tar >V_me)
                MSS = MSSCalculate( V_tar,V_me,V_obj,T_long,Tc,0 ,T_adj);

            elseif (V_obj >= V_me)&&(V_me >V_tar)
                MSS = MSSCalculate( V_tar,V_me,V_obj,T_long,Tc,0 ,T_adj);

            elseif (V_me >= V_obj)&&(V_obj >= V_tar)
                MSSTemp1 = 0;  
                MSSTemp2 = MSSCalculate( V_tar,V_me,V_obj,T_long,Tc,0 ,T_adj);
                MSS = max(MSSTemp1,MSSTemp2);  

            elseif (V_obj <= V_tar)&&(V_tar < V_me)
                MSS = 0;

            elseif (V_obj <= V_me)&&(V_me < V_tar)
                MSS = 0;

            elseif (V_me <= V_obj)&&(V_obj <= V_tar)
                MSS = MSSCalculate( V_tar,V_me,V_obj,T_long,T_max,0 ,T_adj);           
            else
                %Nothing
                MSS = 255;
            end  
        end
    end
end

function MSS = MSSLdJudgment( V_tar,V_me,V_obj,T_long,Tc,T_lat,T_adj )
%UNTITLED5 Summary of this function goes here
%   Detailed explanation goes here

    if abs(V_me-V_tar)<1e-5
    
        if V_me>V_obj
            MSS = (V_me-V_obj)*(T_lat+T_adj);
        else
            MSS = (V_me-V_obj)*(T_adj+Tc);
        end

    else
        T_max = (V_obj - V_me)/(V_tar - V_me)*T_long;
        MSSTemp1 = 0;
        MSSTemp2 = 0;

        if Tc < T_long
            if (V_obj >= V_tar)&&(V_tar >V_me)
                MSS = MSSCalculate( V_tar,V_me,V_obj,T_long,Tc,1 ,T_adj);

            elseif (V_obj >= V_me)&&(V_me >V_tar)
                MSS = MSSCalculate( V_tar,V_me,V_obj,T_long,Tc,1 ,T_adj);

            elseif (V_me >= V_obj)&&(V_obj >= V_tar)
                if Tc > T_max
                    MSS = MSSCalculate( V_tar,V_me,V_obj,T_long,Tc,1 ,T_adj);
                else
                    % Tc < T_max
                    MSS = MSSCalculate( V_tar,V_me,V_obj,T_long,T_max,1 ,T_adj);            
                end

            elseif (V_obj <= V_tar)&&(V_tar < V_me)
                MSS = MSSCalculate( V_tar,V_me,V_obj,T_long,T_lat,1 ,T_adj);

            elseif (V_obj <= V_me)&&(V_me < V_tar)
                MSS = MSSCalculate( V_tar,V_me,V_obj,T_long,T_lat,1 ,T_adj);

            elseif (V_me <= V_obj)&&(V_obj <= V_tar)
                MSSTemp1 = MSSCalculate( V_tar,V_me,V_obj,T_long,T_lat,1 ,T_adj);  
                MSSTemp2 = MSSCalculate( V_tar,V_me,V_obj,T_long,Tc,1 ,T_adj);
                MSS = max(MSSTemp1,MSSTemp2);

            else
                %Nothing
                MSS = 255;
            end    
        else
            % Tc > T_long
            if V_obj > V_tar
                MSS = MSSCalculate( V_tar,V_me,V_obj,T_long,Tc,1 );

            else
                MSS = MSSCalculate( V_tar,V_me,V_obj,T_long,T_lat,1 );

            end    
        end
    end
end

function MSS = MSSLoJudgment( V_tar,V_me,V_obj,T_long,Tc,T_lat,T_adj )
%UNTITLED5 Summary of this function goes here
%   Detailed explanation goes here
    if abs(V_me-V_tar)<1e-5
        if V_me>V_obj
            MSS = (V_me-V_obj)*(Tc+T_adj);
        else
            MSS = 0;
        end
    else
        T_max = (V_obj - V_me)/(V_tar - V_me)*T_long;
        MSSTemp1 = 0;
        MSSTemp2 = 0;

        if Tc < T_long
            if (V_obj >= V_tar)&&(V_tar >V_me)
                %MSS = MSSCalculate( V_tar,V_me,V_obj,T_long,0,1 );
                MSS = 0;
            elseif (V_obj >= V_me)&&(V_me >V_tar)
                %MSS = MSSCalculate( V_tar,V_me,V_obj,T_long,0,1 );
                MSS = 0;
            elseif (V_me >= V_obj)&&(V_obj >= V_tar)
                if Tc > T_max
                    MSS = MSSCalculate( V_tar,V_me,V_obj,T_long,T_max,1 ,T_adj);
                else
                    % Tc < T_max
                    MSS = MSSCalculate( V_tar,V_me,V_obj,T_long,Tc,1 ,T_adj);            
                end

            elseif (V_obj <= V_tar)&&(V_tar < V_me)
                MSS = MSSCalculate( V_tar,V_me,V_obj,T_long,Tc,1 ,T_adj);

            elseif (V_obj <= V_me)&&(V_me < V_tar)
                MSS = MSSCalculate( V_tar,V_me,V_obj,T_long,Tc,1 ,T_adj);

            elseif (V_me <= V_obj)&&(V_obj <= V_tar)
                if Tc < 2*T_max
                    %MSS = MSSCalculate( V_tar,V_me,V_obj,T_long,0,1 );              
                    MSS = 0;
                else 
                    MSS = MSSCalculate( V_tar,V_me,V_obj,T_long,Tc,1 ,T_adj);
                end            
            else
                %Nothing
                MSS = 255;
            end    
        else
            % Tc > T_long
            if (V_obj >= V_tar)&&(V_tar >V_me)
                %MSS = MSSCalculate( V_tar,V_me,V_obj,T_long,0,1 );
                MSS = 0;
            elseif (V_obj >= V_me)&&(V_me >V_tar)
                %MSS = MSSCalculate( V_tar,V_me,V_obj,T_long,0,1 );
                MSS = 0;
            elseif (V_me >= V_obj)&&(V_obj >= V_tar)
                MSS = MSSCalculate( V_tar,V_me,V_obj,T_long,T_max,1 ,T_adj);

            elseif (V_obj <= V_tar)&&(V_tar < V_me)
                MSS = MSSCalculate( V_tar,V_me,V_obj,T_long,Tc,1 ,T_adj);

            elseif (V_obj <= V_me)&&(V_me < V_tar)
                MSS = MSSCalculate( V_tar,V_me,V_obj,T_long,Tc,1 ,T_adj);

            elseif (V_me <= V_obj)&&(V_obj <= V_tar)
                MSSTemp1 = 0;  
                MSSTemp2 = MSSCalculate( V_tar,V_me,V_obj,T_long,Tc,1 ,T_adj);
                MSS = max(MSSTemp1,MSSTemp2);           
            else
                %Nothing
                MSS = 255;
            end  
        end
    end
end

function MSS = MSSCalculate( V_tar,V_me,V_obj,T_long,Time2Cal,ObjDirection ,T_adj)
%UNTITLED3 Summary of this function goes here
%   Detailed explanation goes here

%Time2Cal is the time to be calculated
%V_tar is the target of mergeing vehicle
%V_obj is the obstacle object of mergeing vehicle
%ObjDirection is the direction of object
%T_long is the time when longitual vel adjust ends

    if Time2Cal < T_long
        MSS = (V_tar-V_me)/2/T_long*Time2Cal^2-(V_obj-V_me)*Time2Cal;
    else
        MSS = (V_tar-V_me)/2*T_long - (V_obj - V_me)*T_long - (V_obj - V_tar)*Time2Cal;
    end

    if ObjDirection == 1
        %obj is Leading vehicle 
    else
        %obj is Following vehicle
        MSS = (-1)*MSS;
    end
end

function PreGlbVal(x_inIn,y_inIn,angle_inIn,y_outIn,angle_outIn,Info_FdIn,Info_FoIn,Info_LdIn,Info_LoIn,Info_MeIn,X_melimit_In)
    global V_me V L_veh X_me X L_me T_adj H   Y W_veh  W_me Y_me; 
    global Aylimit Axlimit X_melimit k_maxlimit;
    global T_lat  quadsinu2tbl quadcosu2tbl
    global x_in y_in angle_in y_out angle_out 
%     global MSS  Tc AngleTC
    persistent InitFlg
    if isempty(InitFlg)
        InitFlg = 0;
    end
    Aylimit = 10;
    Axlimit = 10;
    X_melimit = X_melimit_In;
    k_maxlimit = 0.2;
    %Accurcy  3 - > 0.005
    Accurcy = 3;
    %lanewidth
    H = 2.5;
    %Time to adjust vel
    T_adj = 0;
    %Time to change lane
    T_lat = 5;
    %Fd Fo Ld Lo, all are considered to be moving in a constant speed
%     Tc = [0,0,0,0]';
    W_veh = [Info_FdIn(5),Info_FoIn(5),Info_LdIn(5),Info_LoIn(5)]';
    L_veh = [Info_FdIn(4),Info_FoIn(4),Info_LdIn(4),Info_LoIn(4)]';
    Y = [Info_FdIn(2),Info_FoIn(2),Info_LdIn(2),Info_LoIn(2)]';
    X = [Info_FdIn(1),Info_FoIn(1),Info_LdIn(1),Info_LoIn(1)]';
    V = [Info_FdIn(3),Info_FoIn(3),Info_LdIn(3),Info_LoIn(3)]';

    X_me = Info_MeIn(1);
    Y_me = Info_MeIn(2);
    V_me = Info_MeIn(3);
    L_me = Info_MeIn(4);
    W_me = Info_MeIn(5);
    
    x_in = x_inIn;y_in = y_inIn;angle_in = angle_inIn;y_out = y_outIn;angle_out = angle_outIn;
    %Time of end of longitu vel modify
%     MSS = [0,0,0,0]';
%     AngleTC = [0,0,0,0]';
    if InitFlg < 1e-1
        quadsinu2tbl = [0;0;0;0;0;1.00000000000000e-05;1.00000000000000e-05;1.00000000000000e-05;2.00000000000000e-05;3.00000000000000e-05;4.00000000000000e-05;6.00000000000000e-05;7.00000000000000e-05;9.00000000000000e-05;0.000110000000000000;0.000140000000000000;0.000170000000000000;0.000200000000000000;0.000240000000000000;0.000290000000000000;0.000330000000000000;0.000390000000000000;0.000440000000000000;0.000510000000000000;0.000580000000000000;0.000650000000000000;0.000730000000000000;0.000820000000000000;0.000910000000000000;0.00102000000000000;0.00112000000000000;0.00124000000000000;0.00137000000000000;0.00150000000000000;0.00164000000000000;0.00179000000000000;0.00194000000000000;0.00211000000000000;0.00229000000000000;0.00247000000000000;0.00267000000000000;0.00287000000000000;0.00309000000000000;0.00331000000000000;0.00355000000000000;0.00380000000000000;0.00405000000000000;0.00433000000000000;0.00461000000000000;0.00490000000000000;0.00521000000000000;0.00553000000000000;0.00586000000000000;0.00620000000000000;0.00656000000000000;0.00693000000000000;0.00731000000000000;0.00771000000000000;0.00813000000000000;0.00855000000000000;0.00899000000000000;0.00945000000000000;0.00992000000000000;0.0104100000000000;0.0109100000000000;0.0114300000000000;0.0119700000000000;0.0125200000000000;0.0130900000000000;0.0136700000000000;0.0142800000000000;0.0149000000000000;0.0155300000000000;0.0161900000000000;0.0168600000000000;0.0175500000000000;0.0182600000000000;0.0189900000000000;0.0197400000000000;0.0205100000000000;0.0212900000000000;0.0221000000000000;0.0229300000000000;0.0237700000000000;0.0246400000000000;0.0255300000000000;0.0264400000000000;0.0273700000000000;0.0283200000000000;0.0292900000000000;0.0302900000000000;0.0313000000000000;0.0323400000000000;0.0334000000000000;0.0344900000000000;0.0355900000000000;0.0367200000000000;0.0378800000000000;0.0390600000000000;0.0402600000000000;0.0414800000000000;0.0427300000000000;0.0440000000000000;0.0453000000000000;0.0466300000000000;0.0479700000000000;0.0493500000000000;0.0507500000000000;0.0521700000000000;0.0536200000000000;0.0551000000000000;0.0566000000000000;0.0581300000000000;0.0596800000000000;0.0612700000000000;0.0628800000000000;0.0645100000000000;0.0661800000000000;0.0678700000000000;0.0695900000000000;0.0713400000000000;0.0731100000000000;0.0749200000000000;0.0767500000000000;0.0786100000000000;0.0805000000000000;0.0824200000000000;0.0843600000000000;0.0863400000000000;0.0883500000000000;0.0903800000000000;0.0924500000000000;0.0945400000000000;0.0966700000000000;0.0988200000000000;0.101010000000000;0.103220000000000;0.105470000000000;0.107740000000000;0.110050000000000;0.112390000000000;0.114760000000000;0.117160000000000;0.119590000000000;0.122050000000000;0.124540000000000;0.127070000000000;0.129620000000000;0.132210000000000;0.134830000000000;0.137480000000000;0.140160000000000;0.142880000000000;0.145620000000000;0.148400000000000;0.151210000000000;0.154050000000000;0.156920000000000;0.159830000000000;0.162770000000000;0.165740000000000;0.168740000000000;0.171770000000000;0.174840000000000;0.177940000000000;0.181070000000000;0.184230000000000;0.187430000000000;0.190650000000000;0.193910000000000;0.197200000000000;0.200520000000000;0.203880000000000;0.207260000000000;0.210680000000000;0.214130000000000;0.217610000000000;0.221120000000000;0.224670000000000;0.228240000000000;0.231850000000000;0.235480000000000;0.239150000000000;0.242850000000000;0.246580000000000;0.250340000000000;0.254130000000000;0.257950000000000;0.261800000000000;0.265680000000000;0.269590000000000;0.273530000000000;0.277500000000000;0.281490000000000;0.285520000000000;0.289570000000000;0.293660000000000;0.297770000000000;0.301910000000000;0.306070000000000;0.310270000000000;0.314490000000000;0.318740000000000;0.323010000000000;0.327310000000000;0.331640000000000;0.335990000000000;0.340360000000000;0.344770000000000;0.349190000000000;0.353640000000000;0.358110000000000;0.362610000000000;0.367130000000000;0.371670000000000;0.376240000000000;0.380820000000000;0.385430000000000;0.3900600000
00000;0.394710000000000;0.399380000000000;0.404060000000000;0.408770000000000;0.413500000000000;0.418240000000000;0.423000000000000;0.427780000000000;0.432570000000000;0.437380000000000;0.442200000000000;0.447040000000000;0.451900000000000;0.456760000000000;0.461640000000000;0.466540000000000;0.471440000000000;0.476360000000000;0.481280000000000;0.486220000000000;0.491160000000000;0.496120000000000;0.501080000000000;0.506050000000000;0.511020000000000;0.516000000000000;0.520990000000000;0.525980000000000;0.530970000000000;0.535960000000000;0.540960000000000;0.545960000000000;0.550960000000000;0.555960000000000;0.560960000000000;0.565960000000000;0.570950000000000;0.575940000000000;0.580930000000000;0.585910000000000;0.590880000000000;0.595850000000000;0.600810000000000;0.605770000000000;0.610710000000000;0.615640000000000;0.620560000000000;0.625470000000000;0.630360000000000;0.635250000000000;0.640110000000000;0.644960000000000;0.649800000000000;0.654610000000000;0.659410000000000;0.664190000000000;0.668950000000000;0.673680000000000;0.678390000000000;0.683080000000000;0.687750000000000;0.692390000000000;0.697000000000000;0.701580000000000;0.706140000000000;0.710670000000000;0.715160000000000;0.719630000000000;0.724060000000000;0.728460000000000;0.732820000000000;0.737150000000000;0.741440000000000;0.745700000000000;0.749910000000000;0.754080000000000;0.758220000000000;0.762310000000000;0.766360000000000;0.770360000000000;0.774320000000000;0.778240000000000;0.782100000000000;0.785920000000000;0.789690000000000;0.793410000000000;0.797080000000000;0.800690000000000;0.804260000000000;0.807770000000000;0.811220000000000;0.814610000000000;0.817950000000000;0.821240000000000;0.824460000000000;0.827620000000000;0.830720000000000;0.833760000000000;0.836730000000000;0.839640000000000;0.842490000000000;0.845270000000000;0.847980000000000;0.850630000000000;0.853200000000000;0.855710000000000;0.858150000000000;0.860510000000000;0.862810000000000;0.865030000000000;0.867170000000000;0.869250000000000;0.871240000000000;0.873160000000000;0.875010000000000;0.876770000000000;0.878460000000000;0.880070000000000;0.881600000000000;0.883050000000000;0.884420000000000;0.885700000000000;0.886910000000000;0.888030000000000;0.889060000000000;0.890020000000000;0.890880000000000;0.891670000000000;0.892370000000000;0.892980000000000;0.893500000000000;0.893940000000000;0.894290000000000;0.894560000000000;0.894730000000000;0.894820000000000];
        quadcosu2tbl = [0;0.00500000000000000;0.0100000000000000;0.0150000000000000;0.0200000000000000;0.0250000000000000;0.0300000000000000;0.0350000000000000;0.0400000000000000;0.0450000000000000;0.0500000000000000;0.0550000000000000;0.0600000000000000;0.0650000000000000;0.0700000000000000;0.0750000000000000;0.0800000000000000;0.0850000000000000;0.0900000000000000;0.0950000000000000;0.100000000000000;0.105000000000000;0.110000000000000;0.115000000000000;0.120000000000000;0.125000000000000;0.130000000000000;0.135000000000000;0.139990000000000;0.144990000000000;0.149990000000000;0.154990000000000;0.159990000000000;0.164990000000000;0.169990000000000;0.174980000000000;0.179980000000000;0.184980000000000;0.189980000000000;0.194970000000000;0.199970000000000;0.204960000000000;0.209960000000000;0.214950000000000;0.219950000000000;0.224940000000000;0.229940000000000;0.234930000000000;0.239920000000000;0.244910000000000;0.249900000000000;0.254890000000000;0.259880000000000;0.264870000000000;0.269860000000000;0.274840000000000;0.279830000000000;0.284810000000000;0.289790000000000;0.294780000000000;0.299760000000000;0.304740000000000;0.309710000000000;0.314690000000000;0.319660000000000;0.324640000000000;0.329610000000000;0.334580000000000;0.339550000000000;0.344510000000000;0.349480000000000;0.354440000000000;0.359400000000000;0.364350000000000;0.369310000000000;0.374260000000000;0.379210000000000;0.384150000000000;0.389100000000000;0.394040000000000;0.398980000000000;0.403910000000000;0.408840000000000;0.413770000000000;0.418690000000000;0.423620000000000;0.428530000000000;0.433450000000000;0.438350000000000;0.443260000000000;0.448160000000000;0.453050000000000;0.457940000000000;0.462830000000000;0.467710000000000;0.472590000000000;0.477460000000000;0.482320000000000;0.487180000000000;0.492040000000000;0.496880000000000;0.501730000000000;0.506560000000000;0.511390000000000;0.516210000000000;0.521030000000000;0.525830000000000;0.530630000000000;0.535430000000000;0.540210000000000;0.544990000000000;0.549760000000000;0.554520000000000;0.559270000000000;0.564010000000000;0.568750000000000;0.573470000000000;0.578190000000000;0.582890000000000;0.587590000000000;0.592270000000000;0.596940000000000;0.601610000000000;0.606260000000000;0.610900000000000;0.615530000000000;0.620150000000000;0.624750000000000;0.629350000000000;0.633930000000000;0.638490000000000;0.643050000000000;0.647590000000000;0.652110000000000;0.656620000000000;0.661120000000000;0.665600000000000;0.670070000000000;0.674520000000000;0.678960000000000;0.683380000000000;0.687780000000000;0.692170000000000;0.696540000000000;0.700890000000000;0.705220000000000;0.709540000000000;0.713840000000000;0.718120000000000;0.722380000000000;0.726610000000000;0.730830000000000;0.735030000000000;0.739210000000000;0.743370000000000;0.747500000000000;0.751620000000000;0.755710000000000;0.759780000000000;0.763830000000000;0.767850000000000;0.771850000000000;0.775820000000000;0.779770000000000;0.783690000000000;0.787590000000000;0.791470000000000;0.795310000000000;0.799130000000000;0.802920000000000;0.806690000000000;0.810430000000000;0.814130000000000;0.817810000000000;0.821460000000000;0.825080000000000;0.828670000000000;0.832230000000000;0.835760000000000;0.839250000000000;0.842720000000000;0.846150000000000;0.849550000000000;0.852910000000000;0.856240000000000;0.859540000000000;0.862800000000000;0.866030000000000;0.869220000000000;0.872370000000000;0.875490000000000;0.878570000000000;0.881610000000000;0.884610000000000;0.887580000000000;0.890500000000000;0.893390000000000;0.896230000000000;0.899040000000000;0.901800000000000;0.904520000000000;0.907200000000000;0.909840000000000;0.912440000000000;0.914990000000000;0.917500000000000;0.919960000000000;0.922380000000000;0.924750000000000;0.927080000000000;0.929360000000000;0.931590000000000;0.933780000000000;0.935910000000000;0.938000000000000;0.940040000000000;0.942040000000000;0.943980000000000;0.945870000000000;0.947710000000000;0.949500000000000;0.951240000000000;0.952930000000000;0.954570000000000;0.956150000000000;0.957680000000
000;0.959150000000000;0.960570000000000;0.961940000000000;0.963250000000000;0.964510000000000;0.965710000000000;0.966850000000000;0.967940000000000;0.968970000000000;0.969950000000000;0.970860000000000;0.971720000000000;0.972520000000000;0.973260000000000;0.973940000000000;0.974570000000000;0.975130000000000;0.975630000000000;0.976070000000000;0.976450000000000;0.976770000000000;0.977030000000000;0.977230000000000;0.977370000000000;0.977440000000000;0.977450000000000;0.977400000000000;0.977280000000000;0.977100000000000;0.976860000000000;0.976560000000000;0.976190000000000;0.975750000000000;0.975250000000000;0.974690000000000;0.974060000000000;0.973370000000000;0.972610000000000;0.971790000000000;0.970910000000000;0.969960000000000;0.968940000000000;0.967860000000000;0.966710000000000;0.965500000000000;0.964220000000000;0.962880000000000;0.961470000000000;0.959990000000000;0.958450000000000;0.956850000000000;0.955180000000000;0.953440000000000;0.951640000000000;0.949780000000000;0.947850000000000;0.945860000000000;0.943800000000000;0.941670000000000;0.939490000000000;0.937240000000000;0.934920000000000;0.932540000000000;0.930100000000000;0.927600000000000;0.925030000000000;0.922400000000000;0.919710000000000;0.916960000000000;0.914150000000000;0.911280000000000;0.908340000000000;0.905350000000000;0.902300000000000;0.899180000000000;0.896010000000000;0.892790000000000;0.889500000000000;0.886160000000000;0.882760000000000;0.879310000000000;0.875800000000000;0.872240000000000;0.868620000000000;0.864950000000000;0.861230000000000;0.857460000000000;0.853630000000000;0.849760000000000;0.845840000000000;0.841870000000000;0.837850000000000;0.833780000000000;0.829670000000000;0.825520000000000;0.821320000000000;0.817070000000000;0.812790000000000;0.808460000000000;0.804100000000000;0.799690000000000;0.795250000000000;0.790770000000000;0.786250000000000;0.781700000000000;0.777120000000000;0.772500000000000;0.767860000000000;0.763180000000000;0.758470000000000;0.753740000000000;0.748980000000000;0.744190000000000;0.739380000000000;0.734550000000000;0.729700000000000;0.724830000000000;0.719930000000000;0.715030000000000;0.710100000000000;0.705160000000000;0.700210000000000;0.695250000000000;0.690280000000000;0.685300000000000;0.680310000000000;0.675320000000000;0.670320000000000;0.665320000000000];
        InitFlg = 1;          
    end
end
